simulink model "Diff_PlausPrtTrq"  (R2016b)
settings: configuration reference "CodeGenConfigSet" (kept outside this file)
values from neighbouring files (symbols this model uses):
  Diff_dtrqRmpPNeg_C = Calibration.Parameter    [init_Diff_PlausPrtTrq.m]    (also in init_Diff_PlausPrtTrq_SIL.m = Simulink.Parameter)
  Diff_dtrqRmpPPos_C = Calibration.Parameter    [init_Diff_PlausPrtTrq.m]    (also in init_Diff_PlausPrtTrq_SIL.m = Simulink.Parameter)
  Diff_trqPrtErrLim_C = Calibration.Parameter    [init_Diff_PlausPrtTrq.m]    (also in init_Diff_PlausPrtTrq_SIL.m = Simulink.Parameter)
  DiffIO_trqPrtDfftl_C = Calibration.Parameter    [init_Diff_PlausPrtTrq.m]    (also in init_Diff_PlausPrtTrq_SIL.m = Simulink.Parameter)
undefined symbols (not defined in the file or in its folder): Diff_PlausPrtTrq_DT
libraries: CXLib x3
settings Model: Creator=Administrator  LastModifiedBy=Wollf
settings ConfigSetRef: SourceLocation=Base Workspace

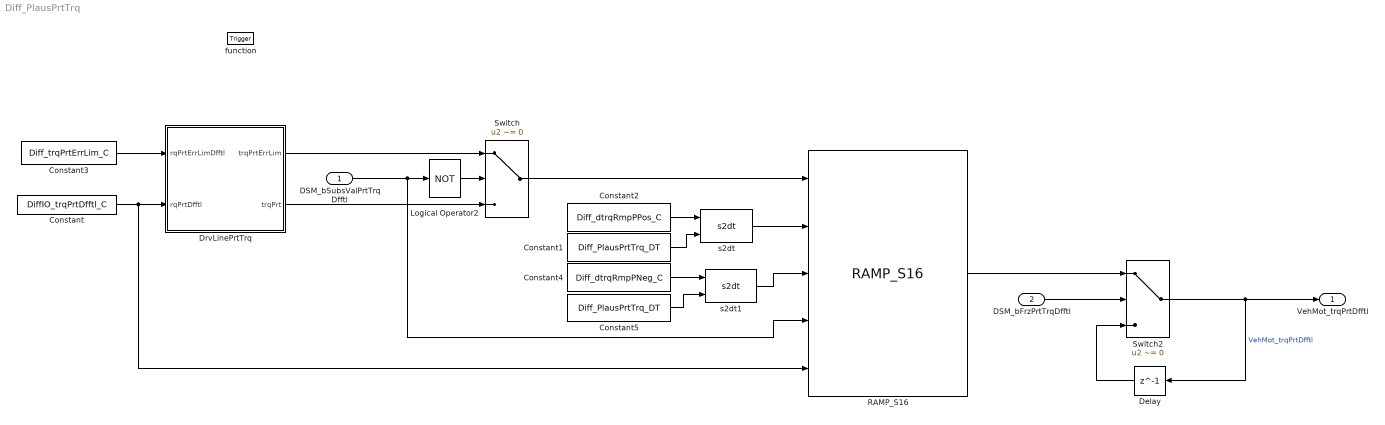
== system Diff_PlausPrtTrq ==
  DSM_bSubsValPrtTrqDfftl : Inport  Description=Status of FId_SubsValPrtTrqDfftl  OutMin=0  OutMax=1  OutDataTypeStr=boolean
  DSM_bFrzPrtTrqDfftl : Inport  Description=Status of FId_FrzPrtTrqDfftl  Port=2  OutMin=0  OutMax=1  OutDataTypeStr=boolean
  function : TriggerPort  TriggerType=function-call  VariantControl=Variant
  Constant : Constant  Value=DiffIO_trqPrtDfftl_C
  Constant1 : Constant  Value=Diff_PlausPrtTrq_DT  OutDataTypeStr=Inherit: Inherit via back propagation
  Constant2 : Constant  Value=Diff_dtrqRmpPPos_C
  Constant3 : Constant  Value=Diff_trqPrtErrLim_C
  Constant4 : Constant  Value=Diff_dtrqRmpPNeg_C
  Constant5 : Constant  Value=Diff_PlausPrtTrq_DT  OutDataTypeStr=Inherit: Inherit via back propagation
  Delay : Delay  DelayLength=1  InitialCondition=0
  DrvLinePrtTrq : Subsystem
  Logical Operator2 : Logic  Operator=NOT  OutDataTypeStr=boolean
  RAMP_S16 : CXLib/RAMP_S16
  Switch : Switch  Criteria=u2 ~= 0  InputSameDT=on
  Switch2 : Switch  Criteria=u2 ~= 0  InputSameDT=on
  s2dt : CXLib/s2dt
  s2dt1 : CXLib/s2dt
  VehMot_trqPrtDfftl : Outport  Tag=Nm  Description=Differential protection torque  OutMin=-3000  OutMax=3000  OutDataTypeStr=Trq_Nm
  wires:
  DSM_bSubsValPrtTrqDfftl/1 -> Logical Operator2/1, RAMP_S16/4
  RAMP_S16/1 -> Switch2/1
  DSM_bFrzPrtTrqDfftl/1 -> Switch2/2
  Constant3/1 -> DrvLinePrtTrq/1(rqPrtErrLimDfftl)
  DrvLinePrtTrq/1(trqPrtErrLim) -> Switch/1
  DrvLinePrtTrq/2(trqPrt) -> Switch/3
  Switch/1 -> RAMP_S16/1
  Constant/1 -> RAMP_S16/5, DrvLinePrtTrq/2(rqPrtDfftl)
  Switch2/1 -> Delay/1, VehMot_trqPrtDfftl/1  "VehMot_trqPrtDfftl"
  Delay/1 -> Switch2/3
  Logical Operator2/1 -> Switch/2
  Constant2/1 -> s2dt/1
  s2dt/1 -> RAMP_S16/2
  s2dt1/1 -> RAMP_S16/3
  Constant4/1 -> s2dt1/1
  Constant1/1 -> s2dt/2
  Constant5/1 -> s2dt1/2

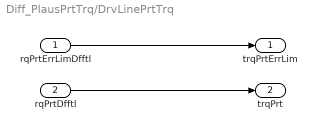
== system Diff_PlausPrtTrq/DrvLinePrtTrq ==
  rqPrtErrLimDfftl : Inport
  rqPrtDfftl : Inport  Port=2
  trqPrtErrLim : Outport
  trqPrt : Outport  Port=2
  wires:
  rqPrtDfftl/1 -> trqPrt/1
  rqPrtErrLimDfftl/1 -> trqPrtErrLim/1
